simulink model "my_simulation"  (R2024b)
settings: Solver=VariableStepAuto  StartTime=0.0  StopTime=10.0  RelTol=1e-3
undefined symbols (not defined in the file): DiscIntNeverNeededParam
settings Model: Creator=xinxing  LastModifiedBy=xinxing

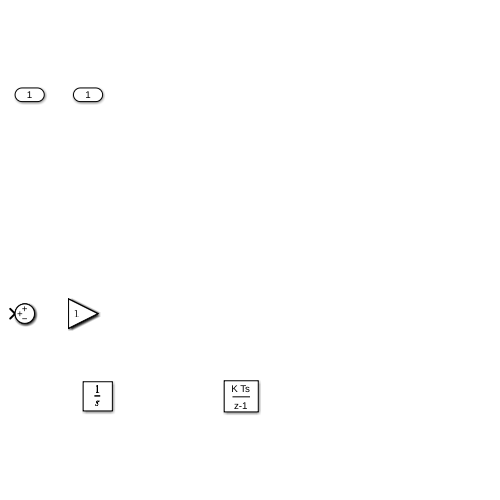
[thumbnail: Simulink's stored preview of the top-level diagram]
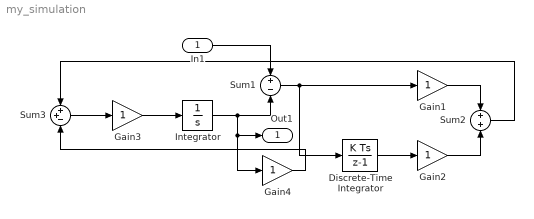
== system my_simulation ==
  In1 : Inport
  Discrete-Time Integrator : DiscreteIntegrator  SampleTime=-1  ICPrevOutput=DiscIntNeverNeededParam  ICPrevScaledInput=DiscIntNeverNeededParam
  Gain{1..4} (4 alike) : Gain
  Integrator : Integrator
  Sum1 : Sum  Inputs=+-
  Sum2 : Sum
  Sum3 : Sum  Inputs=++-
  Out1 : Outport
  wires:
  Sum2/1 -> Sum3/1
  Gain2/1 -> Sum2/2
  Gain1/1 -> Sum2/1
  Discrete-Time Integrator/1 -> Gain2/1
  Gain4/1 -> Sum3/3
  Sum1/1 -> Discrete-Time Integrator/1, Gain1/1
  In1/1 -> Sum1/1
  Gain3/1 -> Integrator/1
  Integrator/1 -> Out1/1, Gain4/1, Sum1/2
  Sum3/1 -> Gain3/1
